simulink model "PlantaV4_2"  (R2021a)
settings: Solver=VariableStepAuto  StartTime=0.0  StopTime=60  MaxStep=1e-2  RelTol=1e-3
values from neighbouring files (symbols this model uses):
  alfahmax = ((2*ahmax)/(rhd))    (= 2)    [valoresPlanta_29_9_24.m]    (also in valoresPlanta_V3.m; valoresPlanta_v4.m)
  alfatmax = atmax/rtd    (= 1.6)    [valoresPlanta_29_9_24.m]    (also in valoresPlanta_V3.m; valoresPlanta_v4.m)
  atmax = 0.8    [valoresPlanta_29_9_24.m]    (also in valoresPlanta_V3.m; valoresPlanta_v4.m)
  ax_max = 0.8    [valoresPlanta_29_9_24.m]    (also in valoresPlanta_v4.m)
  ay_max = 0.75    [valoresPlanta_29_9_24.m]    (also in valoresPlanta_v4.m)
  bh_eq = bhm*ih^2+bhd    (= 8720)    [Valores.m]    (also in Valores_1.m; valoresPlanta.m; valoresPlanta_29_9_24.m; valoresPlanta_V3.m)
  bhb = 1e8    (= 100000000)    [Valores.m]    (also in Valores_1.m; valoresPlanta.m; valoresPlanta_29_9_24.m; valoresPlanta_V3.m)
  bhEb = 2.2e9    (= 2200000000)    [Valores.m]    (also in Valores_1.m; valoresPlanta.m; valoresPlanta_29_9_24.m; valoresPlanta_V3.m)
  bt = 90.0    (= 90)    [Valores.m]    (also in Valores_1.m; valoresPlanta.m; valoresPlanta_29_9_24.m; valoresPlanta_V3.m)
  bt_eq = btd+(btm*(it^2))    (= 5401.8)    [valoresPlanta.m]    (also in valoresPlanta_29_9_24.m; valoresPlanta_V3.m; valoresPlanta_v4.m)
  btw = 3.0e3    (= 3000)    [Valores.m]    (also in Valores_1.m; valoresPlanta.m; valoresPlanta_29_9_24.m; valoresPlanta_V3.m)
  bwu = 150    [Valores.m]    (also in Valores_1.m; valoresPlanta.m; valoresPlanta_29_9_24.m; valoresPlanta_V3.m)
  g = 9.80665    [Valores.m]    (also in Valores_1.m; valoresPlanta.m; valoresPlanta_29_9_24.m; valoresPlanta_V3.m)
  hMax = 10    [Valores_1.m]    (also in valoresPlanta.m; valoresPlanta_V3.m; valoresPlanta_v4.m)
  ih = 22    [Valores.m]    (also in Valores_1.m; valoresPlanta.m; valoresPlanta_29_9_24.m; valoresPlanta_V3.m)
  it = 30    [Valores.m]    (also in Valores_1.m; valoresPlanta.m; valoresPlanta_29_9_24.m; valoresPlanta_V3.m)
  Jh_eq = Jhm_hb*ih^2+Jhd_hEb    (= 18320)    [Valores.m]    (also in Valores_1.m; valoresPlanta.m; valoresPlanta_29_9_24.m; valoresPlanta_V3.m)
  Jt_eq = Jtd+(Jtm_tb*(it^2))    (= 7500)    [valoresPlanta.m]    (also in valoresPlanta_29_9_24.m; valoresPlanta_V3.m; valoresPlanta_v4.m)
  KDh = Jeq2 * w_posh^3    (= -12245.4404091)    [Valores.m]    (also in Valores_1.m = Jeq2 * w_posh; valoresPlanta.m = Jeq2 * w_posh; valoresPlanta_29_9_24.m = Jh_eq * n * w_posh; valoresPlanta_V3.m = Jeq2 * w_posh)
  KDt = Meq2 * w_post^3    (= -4728.86946035)    [Valores.m]    (also in Valores_1.m = Meq2 * w_post; valoresPlanta.m = Meq2 * w_post; valoresPlanta_29_9_24.m = 10127; valoresPlanta_V3.m = Meq2 * w_post)
  KIh = Jeq2 * w_posh^2    (= 2572.66592082)    [Valores.m]    (also in Valores_1.m = Jeq2 * w_posh^3; valoresPlanta.m = Jeq2 * w_posh^3; valoresPlanta_29_9_24.m = Jh_eq * w_posh^3; valoresPlanta_V3.m = Jeq2 * w_posh^3)
  KIt = Meq2 * w_post^2    (= 1307.690244)    [Valores.m]    (also in Valores_1.m = Meq2 * w_post^3; valoresPlanta.m = Meq2 * w_post^3; valoresPlanta_29_9_24.m = 6809.6; valoresPlanta_V3.m = Meq2 * w_post^3)
  KPh = Jeq2 * w_posh    (= -540.495867769)    [Valores.m]    (also in Valores_1.m = Jeq2 * w_posh^2; valoresPlanta.m = Jeq2 * w_posh^2; valoresPlanta_29_9_24.m = Jh_eq * n * w_posh^2; valoresPlanta_V3.m = Jeq2 * w_posh^2)
  KPt = Meq2 * w_post    (= -361.62)    [Valores.m]    (also in Valores_1.m = Meq2 * w_post^2; valoresPlanta.m = Meq2 * w_post^2; valoresPlanta_29_9_24.m = 14123; valoresPlanta_V3.m = Meq2 * w_post^2)
  Ktw = 4.8e5    (= 480000)    [Valores.m]    (also in Valores_1.m; valoresPlanta.m; valoresPlanta_29_9_24.m; valoresPlanta_V3.m)
  kwu = 2.36e8    (= 236000000)    [Valores.m]    (also in Valores_1.m; valoresPlanta.m; valoresPlanta_29_9_24.m; valoresPlanta_V3.m)
  Mc_max = 5e4    (= 50000)    [Valores.m]    (also in Valores_1.m; valoresPlanta.m; valoresPlanta_29_9_24.m; valoresPlanta_V3.m)
  Mc_min = 2e3    (= 2000)    [Valores.m]    (also in Valores_1.m; valoresPlanta.m; valoresPlanta_29_9_24.m; valoresPlanta_V3.m)
  Meq = Mt+(it^2*Jtm_tb+Jtd)/rtd^2    (= 60000)    [Valores.m]    (also in Valores_1.m; valoresPlanta_29_9_24.m; valoresPlanta_v4.m)
  Ms = 1.5e4    (= 15000)    [Valores.m]    (also in Valores_1.m; valoresPlanta.m; valoresPlanta_29_9_24.m; valoresPlanta_V3.m)
  Mt = 30000    [Valores.m]    (also in Valores_1.m; valoresPlanta.m; valoresPlanta_29_9_24.m; valoresPlanta_V3.m)
  pos = [p0; p1; p2; p3; p4; p5]    [calcularTrayectoria2_prueba.m]    (also in perfilObsaculos.m = puntosTrayectoria(4, 1.5, 20, [-20,0], estado_cont, hy_cont,; puntosTrayectoria.m; valoresPlanta_29_9_24.m = calcularTrayectoria2_prueba(vx_max, vhmax, ax_max, Hc, hx_co; valoresPlanta_v4.m = puntosTrayectoria(4, 1.5, 20, [-20,0], estado_cont, hy_cont,)
  rhd = 0.75    [Valores.m]    (also in Valores_1.m; valoresPlanta.m; valoresPlanta_29_9_24.m; valoresPlanta_V3.m)
  rtd = 0.5    [Valores.m]    (also in Valores_1.m; valoresPlanta.m; valoresPlanta_29_9_24.m; valoresPlanta_V3.m)
  tau_hm = 1e-3    (= 0.001)    [valoresPlanta.m]    (also in valoresPlanta_29_9_24.m; valoresPlanta_V3.m; valoresPlanta_v4.m)
  tau_tm = 1e-3    (= 0.001)    [Valores.m]    (also in Valores_1.m; valoresPlanta.m; valoresPlanta_29_9_24.m; valoresPlanta_V3.m)
  Thb_Max = 5e4    (= 50000)    [Valores.m]    (also in Valores_1.m; valoresPlanta.m; valoresPlanta_29_9_24.m; valoresPlanta_V3.m)
  ThEb_Max = 1.1e6    (= 1100000)    [Valores.m]    (also in Valores_1.m; valoresPlanta.m; valoresPlanta_29_9_24.m; valoresPlanta_V3.m)
  Thm_Max = 2e4    (= 20000)    [Valores.m]    (also in Valores_1.m; valoresPlanta.m; valoresPlanta_29_9_24.m; valoresPlanta_V3.m)
  Ttb_Max = 5e3    (= 5000)    [Valores.m]    (also in Valores_1.m; valoresPlanta.m; valoresPlanta_29_9_24.m; valoresPlanta_V3.m)
  Ttm_Max = 3e3    (= 3000)    [Valores.m]    (also in Valores_1.m; valoresPlanta.m; valoresPlanta_29_9_24.m = 4000; valoresPlanta_V3.m)
  v_x_max = 4    [Valores_1.m]    (also in valoresPlanta.m; valoresPlanta_V3.m = 0.4; valoresPlanta_v4.m)
  Yt0 = 45    [Valores.m]    (also in Valores_1.m; valoresPlanta.m; valoresPlanta_29_9_24.m; valoresPlanta_V3.m)
undefined symbols (not defined in the file or in its folder): sigbuilder_block
libraries: simulink_extras x1
settings Model: Creator=Matias  LastModifiedBy=agustin

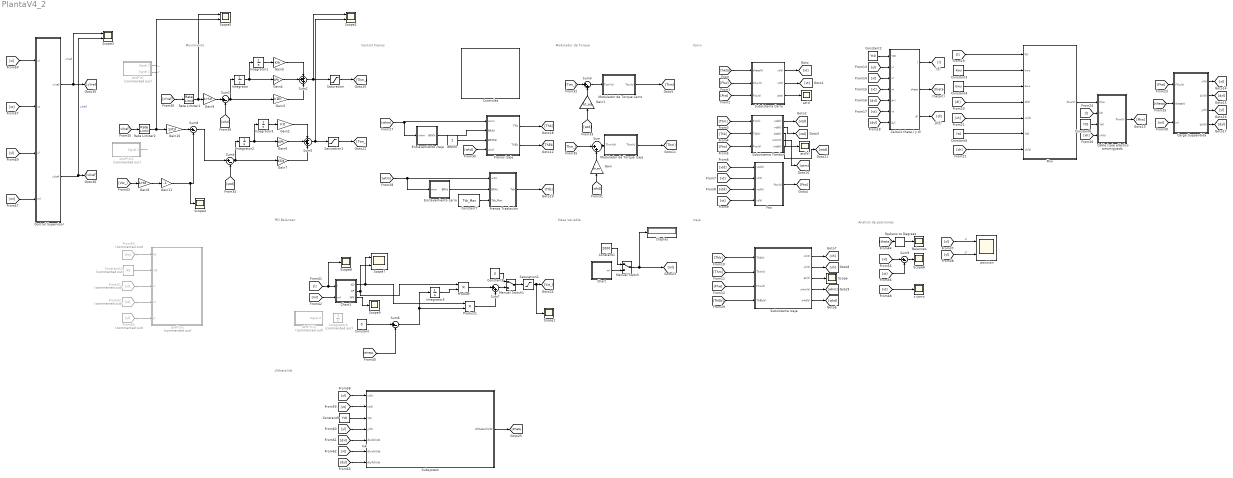
== system PlantaV4_2 ==
  note: d(theta)/dt
  note: Analisis de posiciones
  note: PID Balanceo
  note: Masa Variable
  note: Control Frenos
  note: Izaje
  note: Modulador de Torque
  note: Carro
  note: Movimiento
  In4 : Inport
  BRKhE : Constant
  Balanceo : Scope
  Cable izaje elástico amortiguado : Subsystem
  Calculo theta,l y dl : Subsystem
  Carga Suspendida : Subsystem
  Chart : Stateflow chart  TreatAsAtomicUnit=on
  Chart1 : Stateflow chart  TreatAsAtomicUnit=on
  Constant : Constant  Value=0
  Constant1 : Constant  Value=2000
  Constant12 : Constant  Commented=on  Value=45
  Constant{2,5..6,9} (4 alike) : Constant  Value=Yt0
  Constant3 : Constant  Value=kwu
  Constant4 : Constant  Value=bwu
  Constant7 : Constant  Value=Ttb_Max
  Constant8 : Constant  Value=0
  Control Supervisor : Subsystem
  Controles : Subsystem
  Display : Display
  Enclavamiento carro : Stateflow chart  TreatAsAtomicUnit=on
  Enclavamiento izaje : Stateflow chart  TreatAsAtomicUnit=on
  Fhw : Subsystem
  "Frenos Izaje " : Stateflow chart  TreatAsAtomicUnit=on
  Frenos Traslación : Stateflow chart  TreatAsAtomicUnit=on
  From51 : From  Commented=on  GotoTag=xl
  From52 : From  Commented=on  GotoTag=xt
  From53 : From  Commented=on  GotoTag=hc
  From54 : From  Commented=on  GotoTag=yl
  Ftw : Subsystem
  Gain : Gain  Gain=bh_eq
  Gain1 : Gain  Gain=bt_eq
  Gain10 : Gain  Gain=1/rtd
  Gain11 : Gain  Gain=.1
  Gain2 : Gain  Gain=KIt
  Gain3 : Gain  Gain=KDh
  Gain4 : Gain  Gain=KPh
  Gain5 : Gain  Gain=KIh
  Gain6 : Gain  Gain=KPt
  Gain7 : Gain  Gain=KDt
  Gain8 : Gain  Gain=1/rtd
  Gain9 : Gain  Gain=2/rhd
  Integrator{,1..3,5} (5 alike) : Integrator
  Integrator4 : Integrator  Commented=on
  Manual Switch : ManualSwitch
  Manual Switch1 : ManualSwitch
  Modulador de Torque Carro : Subsystem
  Modulador de Torque Izaje : Subsystem
  Product : Product
  Product1 : Product
  Radians to Degrees : simulink_extras/Transformations/Radians to Degrees
  Rate Limiter1 : RateLimiter  RisingSlewLimit=ay_max  FallingSlewLimit=-ay_max  SampleTimeMode=inherited
  Rate Limiter2 : RateLimiter  RisingSlewLimit=ax_max  FallingSlewLimit=-ax_max  SampleTimeMode=inherited
  Saturation : Saturate  UpperLimit=Thm_Max  LowerLimit=-Thm_Max
  Saturation1 : Saturate  UpperLimit=Ttm_Max  LowerLimit=-Ttm_Max
  Saturation2 : Saturate  UpperLimit=4  LowerLimit=-4
  Scope{,1,4,6,8..9} (6 alike) : Scope
  Scope{2..3,5,7} (4 alike) : Scope  NumInputPorts=2
  Subsistema Carro : Subsystem
  Subsistema Izaje : Subsystem
  Subsistema Tambor : Subsystem
  Subsystem : Subsystem
  Sum : Sum  Inputs=|++
  Sum{1,4,6,8..9} (5 alike) : Sum  Inputs=|+-
  Sum2 : Sum  Inputs=+++
  Sum3 : Sum  Inputs=|++
  Sum5 : Sum  Inputs=+++
  Sum7 : Sum  Inputs=|++
  at(t) : Scope
  atd(t) : Scope
  graficos : Stateflow chart  Commented=on  TreatAsAtomicUnit=on
  posicion : Scope  NumInputPorts=2
  whd*(t) : Subsystem  Tag=STV Subsys  Commented=on  LoadFcn=sigbuilder_block('load');  StartFcn=sigbuilder_block('start');  StopFcn=sigbuilder_block('stop');  ClipboardFcn=sigbuilder_block('clipboard');  mask(Sigbuilder block){tuvar=[0:10]}
      mask help: Simulink:masks:SigbuilderBlock_MD
      mask init:
      | if ~strcmp(get_param(bdroot(gcbh),'SimulationStatus'),'stopped') tuvar = sigbuilder_block('maskInit'); end
      settings: CopyFcn=sigbuilder_block('copy');  DeleteFcn=sigbuilder_block('delete');  ModelCloseFcn=sigbuilder_block('modelClose');  PreSaveFcn=sigbuilder_block('preSave');  PauseFcn=sigbuilder_block('pause');  ContinueFcn=sigbuilder_block('continue');  NameChangeFcn=sigbuilder_block('namechange');  OpenFcn=sigbuilder_block('open',[437.6 153 550.4 359.25 ]);  CloseFcn=sigbuilder_block('close');
      mask Display: plot(0, 0, 100, 100,[2, 2, 32, 32, 2], [68, 8, 8, 68, 68],[32, 2], [38, 38], [32, 19, 2],[53, 60, 44], [32, 17, 17, 2],[16, 16, 31, 31]);txt = getActiveGroup(gcbh);text(2, 100, txt,'verticalAlignment', 'top');
  whd*(t)1 : Subsystem  Tag=STV Subsys  Commented=on  LoadFcn=sigbuilder_block('load');  StartFcn=sigbuilder_block('start');  StopFcn=sigbuilder_block('stop');  ClipboardFcn=sigbuilder_block('clipboard');  mask(Sigbuilder block){tuvar=[0:10]}
      mask help: Simulink:masks:SigbuilderBlock_MD
      mask init:
      | if ~strcmp(get_param(bdroot(gcbh),'SimulationStatus'),'stopped') tuvar = sigbuilder_block('maskInit'); end
      settings: CopyFcn=sigbuilder_block('copy');  DeleteFcn=sigbuilder_block('delete');  ModelCloseFcn=sigbuilder_block('modelClose');  PreSaveFcn=sigbuilder_block('preSave');  PauseFcn=sigbuilder_block('pause');  ContinueFcn=sigbuilder_block('continue');  NameChangeFcn=sigbuilder_block('namechange');  OpenFcn=sigbuilder_block('open',[437.6 199.2 550.4 400 ]);  CloseFcn=sigbuilder_block('close');
      mask Display: plot(0, 0, 100, 100,[2, 2, 32, 32, 2], [68, 8, 8, 68, 68],[32, 2], [38, 38], [32, 19, 2],[53, 60, 44], [32, 17, 17, 2],[16, 16, 31, 31]);txt = getActiveGroup(gcbh);text(2, 100, txt,'verticalAlignment', 'top');
  whd*(t)2 : Subsystem  Tag=STV Subsys  Commented=on  LoadFcn=sigbuilder_block('load');  StartFcn=sigbuilder_block('start');  StopFcn=sigbuilder_block('stop');  ClipboardFcn=sigbuilder_block('clipboard');  mask(Sigbuilder block){tuvar=[0:10]}
      mask help: Simulink:masks:SigbuilderBlock_MD
      mask init:
      | if ~strcmp(get_param(bdroot(gcbh),'SimulationStatus'),'stopped') tuvar = sigbuilder_block('maskInit'); end
      settings: CopyFcn=sigbuilder_block('copy');  DeleteFcn=sigbuilder_block('delete');  ModelCloseFcn=sigbuilder_block('modelClose');  PreSaveFcn=sigbuilder_block('preSave');  PauseFcn=sigbuilder_block('pause');  ContinueFcn=sigbuilder_block('continue');  NameChangeFcn=sigbuilder_block('namechange');  OpenFcn=sigbuilder_block('open',[437.6 153 550.4 359.25 ]);  CloseFcn=sigbuilder_block('close');
      mask Display: plot(0, 0, 100, 100,[2, 2, 32, 32, 2], [68, 8, 8, 68, 68],[32, 2], [38, 38], [32, 19, 2],[53, 60, 44], [32, 17, 17, 2],[16, 16, 31, 31]);txt = getActiveGroup(gcbh);text(2, 100, txt,'verticalAlignment', 'top');
  x carro : Scope
  wires:
  Subsistema Tambor/1(xtd(t)) -> [xtd]
  Subsistema Tambor/2(vtd(t)) -> [vtd]
  Subsistema Carro/1(xt(t)) -> [xt]
  Subsistema Carro/2(vt(t)) -> [vt]
  Subsistema Carro/3(at(t)) -> at(t)/1
  Subsistema Tambor/3(atd(t)) -> atd(t)/1
  [Ttb] -> Subsistema Tambor/2(Ttb(t))
  [Ttm] -> Subsistema Tambor/1(Tm(t))
  [Ftw] -> Subsistema Carro/3(Ftw(t))
  [Fhw] -> Subsistema Carro/2(Fhw(t))
  [theta] -> Subsistema Carro/1(theta(t))
  [Ftw] -> Subsistema Tambor/3(Ftw(t))
  Ftw/1(Ftw(t)) -> [Ftw]
  [xtd] -> Ftw/1(xtd(t))
  [xt] -> Ftw/2(xt(t))
  [vtd] -> Ftw/3(vtd(t))
  [vt] -> Ftw/4(vt(t))
  Modulador de Torque Carro/1(Ttm(t)) -> [Ttm]
  [Thm] -> Subsistema Izaje/2(Thm(t))
  [Thb] -> Subsistema Izaje/1(Thb(t))
  [Fhw] -> Subsistema Izaje/3(Fhw(t))
  Subsistema Izaje/1(xh(t)) -> [xh]
  Subsistema Izaje/2(vh(t)) -> [vh]
  Subsistema Izaje/3(ah(t)) -> Scope/1
  Subsistema Izaje/4(whm(t)) -> [whm]
  Subsistema Tambor/4(wtm(t)) -> [wtm]
  Modulador de Torque Izaje/1(Thm(t)) -> [Thm]
  [dxl] -> Calculo theta,l y dl/5(dxl)
  Constant2/1 -> Calculo theta,l y dl/1(Yt0)
  [yl] -> Calculo theta,l y dl/2(yl)
  Calculo theta,l y dl/3(dl) -> [dl]
  Calculo theta,l y dl/1(l) -> [l]
  [dyl] -> Calculo theta,l y dl/7(dyl)
  [xl] -> Calculo theta,l y dl/3(xl)
  [vt] -> Calculo theta,l y dl/6(vt)
  [xt] -> Calculo theta,l y dl/4(xt)
  Calculo theta,l y dl/2(theta) -> [theta]
  [dl] -> Fhw/4(dl(t))
  [xh] -> Fhw/7(xh(t))
  Constant3/1 -> Fhw/2(kwu)
  [l] -> Fhw/1(l(t))
  Constant5/1 -> Fhw/6(Yt0)
  [vh] -> Fhw/5(vh(t))
  Constant4/1 -> Fhw/3(bwu)
  Fhw/1(Fhw(t)) -> Cable izaje elástico amortiguado/1(Fhw)
  [l] -> Cable izaje elástico amortiguado/2(l(t))
  Constant6/1 -> Cable izaje elástico amortiguado/3(Yt0)
  [xh] -> Cable izaje elástico amortiguado/4(xh(t))
  Cable izaje elástico amortiguado/1(Fhw(t)) -> [Fhw]
  [theta] -> Carga Suspendida/2(theta(t))
  [Fhw] -> Carga Suspendida/1(Fhw(t))
  Carga Suspendida/1(xl(t)) -> [xl]
  Carga Suspendida/4(dyl(t)) -> [dyl]
  Carga Suspendida/3(yl(t)) -> [yl]
  Carga Suspendida/2(dxl(t)) -> [dxl]
  [whm] -> "Frenos Izaje "/1(whm), Enclavamiento izaje/1(whm)
  [wtm] -> Enclavamiento carro/1(wtm), Frenos Traslación/1(wtm)
  Enclavamiento carro/1(BRKt) -> Frenos Traslación/2(BRKt)
  Enclavamiento izaje/1(BRKh) -> "Frenos Izaje "/2(BRKh)
  "Frenos Izaje "/2(ThEb) -> [ThEb]
  Constant7/1 -> Frenos Traslación/3(Ttb_Max)
  BRKhE/1 -> "Frenos Izaje "/3(BRKhE)
  "Frenos Izaje "/1(Thb) -> [Thb]
  Frenos Traslación/1(Ttb) -> [Ttb]
  Subsistema Izaje/5(whd(t)) -> [whd]
  [ThEb] -> Subsistema Izaje/4(ThEb(t))
  [whd] -> "Frenos Izaje "/4(whd)
  [Thm_] -> Sum/1
  Sum/1 -> Modulador de Torque Izaje/1(Thm*(t))
  [whd] -> Gain/1
  Gain/1 -> Sum/2
  Integrator1/1 -> Gain5/1
  Integrator/1 -> Integrator1/1, Gain4/1
  Sum1/1 -> Integrator/1, Gain3/1
  Gain4/1 -> Sum2/2
  Gain5/1 -> Sum2/1
  Gain3/1 -> Sum2/3
  Sum3/1 -> Modulador de Torque Carro/1(Ttm*(t))
  [Ttm_] -> Sum3/1
  Gain1/1 -> Sum3/2
  Subsistema Tambor/5(wtd(t)) -> [wtd]
  [wtd] -> Gain1/1
  Gain7/1 -> Sum5/3
  [wtd] -> Sum4/2
  Gain6/1 -> Sum5/2
  Gain2/1 -> Sum5/1
  Integrator2/1 -> Integrator3/1, Gain6/1
  Sum4/1 -> Gain7/1, Integrator2/1
  Integrator3/1 -> Gain2/1
  [xl] -> posicion/1  "xl"
  [yl] -> posicion/2  "yl"
  [whd] -> Sum1/2
  Manual Switch/1 -> Display/1, [ml]
  [ml] -> Carga Suspendida/3(ml)
  [l] -> Scope8/1, Chart1/1(l)
  [ml] -> Chart1/2(ml)
  Product/1 -> Sum7/1
  Product1/1 -> Sum7/2
  Sum6/1 -> Product1/2, Integrator5/1
  Chart1/1(KD) -> Scope7/1, Product1/1
  Chart1/2(KP) -> Product/1, Scope7/2
  Constant/1 -> Sum6/1
  Sum8/1 -> Sum4/1
  whd*(t)2/1(Signal 2) -> ?
  Sum7/1 -> Manual Switch1/2
  Chart/1(ml) -> Manual Switch/2
  Constant1/1 -> Manual Switch/1
  Constant8/1 -> Manual Switch1/1
  [yl] -> Control Supervisor/3(yl)
  Control Supervisor/2(vXref) -> Scope3/2, [vXref]  "vXref"
  Control Supervisor/1(vYref) -> Scope3/1, [vYref]  "vYref"
  [xl] -> Control Supervisor/1(xl)
  whd*(t)/2(Signal 1) -> ?
  whd*(t)/1(Signal 2) -> ?
  Gain9/1 -> Sum1/1
  Manual Switch1/1 -> Saturation2/1
  [ml] -> Control Supervisor/4(ml)
  Constant12/1 -> graficos/2(Yt0)
  From52/1 -> graficos/4(xt)
  From51/1 -> graficos/3(xl)
  From53/1 -> graficos/1(Hc)
  From54/1 -> graficos/5(yl)
  Sum2/1 -> Saturation/1, Scope2/1
  [xl] -> Sum9/1
  [xt] -> Sum9/2
  Sum9/1 -> Scope6/1
  [xt] -> x carro/1
  Radians to Degrees/1 -> Balanceo/1
  [theta] -> Radians to Degrees/1
  Chart1/3(WN) -> Scope9/1
  [dTheta] -> Sum6/2
  Integrator5/1 -> Product/2
  Gain8/1 -> Gain11/1
  Gain11/1 -> Sum8/2, Scope4/1
  [Vxt_] -> Gain8/1
  Sum5/1 -> Saturation1/1, Scope2/2
  Gain10/1 -> Sum8/1
  [xt] -> Control Supervisor/2(xt)
  [vYref] -> Rate Limiter1/1
  [vXref] -> Rate Limiter2/1
  [dyl] -> Subsystem/7(d(yl(t))/dt)
  [vt] -> Subsystem/6(d(xt(t))/dt)
  [dxl] -> Subsystem/5(d(xl(t))/dt)
  [yl] -> Subsystem/4(yl(t))
  [xt] -> Subsystem/2(xt(t))
  [xl] -> Subsystem/1(xl(t))
  Constant9/1 -> Subsystem/3(Yto)
  Subsystem/1(d(theta(t))/dt) -> [dTheta]
  Rate Limiter2/1 -> Gain10/1, Scope5/2
  Rate Limiter1/1 -> Scope5/1, Gain9/1
  Saturation2/1 -> Scope1/1, [Vxt_]
  Saturation/1 -> [Thm_]
  Saturation1/1 -> [Ttm_]

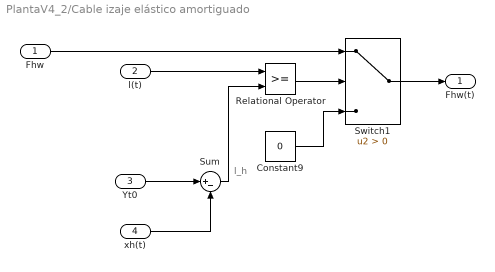
== system PlantaV4_2/Cable izaje elástico amortiguado ==
  note: l_h
  Fhw : Inport
  l(t) : Inport  Port=2
  Yt0 : Inport  Port=3
  xh(t) : Inport  Port=4
  Constant9 : Constant  Value=0
  Relational Operator : RelationalOperator  OutDataTypeStr=boolean  RndMeth=Simplest
  Sum : Sum  Inputs=|+-
  Switch1 : Switch  Criteria=u2 > Threshold
  Fhw(t) : Outport
  wires:
  l(t)/1 -> Relational Operator/1
  Sum/1 -> Relational Operator/2
  Fhw/1 -> Switch1/1
  Yt0/1 -> Sum/1
  Constant9/1 -> Switch1/3
  Relational Operator/1 -> Switch1/2
  xh(t)/1 -> Sum/2
  Switch1/1 -> Fhw(t)/1

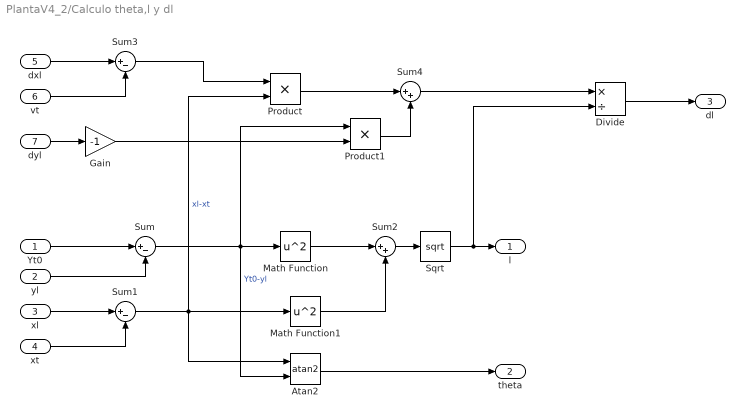
== system PlantaV4_2/Calculo theta,l y dl ==
  Yt0 : Inport
  yl : Inport  Port=2
  xl : Inport  Port=3
  xt : Inport  Port=4
  dxl : Inport  Port=5
  vt : Inport  Port=6
  dyl : Inport  Port=7
  Atan2 : Trigonometry  Operator=atan2
  Divide : Product  Inputs=*/
  Gain : Gain  Gain=-1
  Math Function : Math  Operator=square  SaturateOnIntegerOverflow=on
  Math Function1 : Math  Operator=square  SaturateOnIntegerOverflow=on
  Product : Product
  Product1 : Product
  Sqrt : Sqrt  SaturateOnIntegerOverflow=on
  Sum : Sum  Inputs=|+-
  Sum1 : Sum  Inputs=|+-
  Sum2 : Sum  Inputs=|++
  Sum3 : Sum  Inputs=|+-
  Sum4 : Sum  Inputs=|++
  l : Outport
  theta : Outport  Port=2
  dl : Outport  Port=3
  wires:
  Yt0/1 -> Sum/1
  yl/1 -> Sum/2
  xl/1 -> Sum1/1
  xt/1 -> Sum1/2
  Atan2/1 -> theta/1
  Sum1/1 -> Product/2, Math Function1/1, Atan2/1  "xl-xt"
  Sum/1 -> Product1/1, Atan2/2, Math Function/1  "Yt0-yl"
  Math Function/1 -> Sum2/1
  Math Function1/1 -> Sum2/2
  Sum2/1 -> Sqrt/1
  Sqrt/1 -> Divide/2, l/1
  dxl/1 -> Sum3/1
  vt/1 -> Sum3/2
  Sum3/1 -> Product/1
  dyl/1 -> Gain/1
  Gain/1 -> Product1/2
  Product/1 -> Sum4/1
  Product1/1 -> Sum4/2
  Sum4/1 -> Divide/1
  Divide/1 -> dl/1

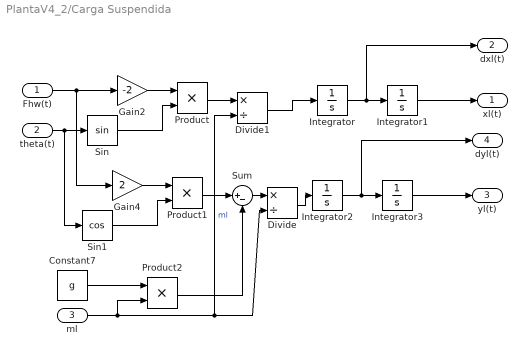
== system PlantaV4_2/Carga Suspendida ==
  Fhw(t) : Inport
  theta(t) : Inport  Port=2
  ml : Inport  Port=3
  Constant7 : Constant  Value=g
  Divide : Product  Inputs=*/
  Divide1 : Product  Inputs=*/
  Gain2 : Gain  Gain=-2
  Gain4 : Gain  Gain=2
  Integrator{,1..3} (4 alike) : Integrator
  Product : Product
  Product1 : Product
  Product2 : Product
  Sin : Trigonometry
  Sin1 : Trigonometry  Operator=cos
  Sum : Sum  Inputs=|+-
  xl(t) : Outport
  dxl(t) : Outport  Port=2
  yl(t) : Outport  Port=3
  dyl(t) : Outport  Port=4
  wires:
  Divide1/1 -> Integrator/1
  theta(t)/1 -> Sin1/1, Sin/1
  Constant7/1 -> Product2/1
  Product2/1 -> Sum/2
  Product/1 -> Divide1/1
  Fhw(t)/1 -> Gain4/1, Gain2/1
  Sum/1 -> Divide/1
  Integrator/1 -> dxl(t)/1, Integrator1/1
  Sin1/1 -> Product1/2
  Gain2/1 -> Product/1
  Product1/1 -> Sum/1
  Sin/1 -> Product/2
  Integrator1/1 -> xl(t)/1
  Integrator2/1 -> dyl(t)/1, Integrator3/1
  Divide/1 -> Integrator2/1
  Gain4/1 -> Product1/1
  Integrator3/1 -> yl(t)/1
  ml/1 -> Divide1/2, Divide/2, Product2/2  "ml"

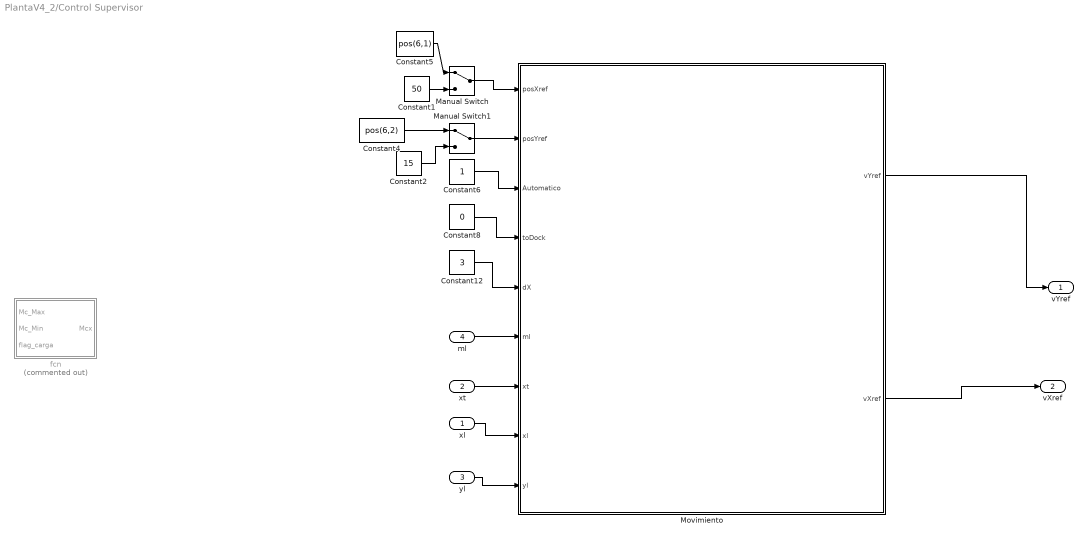
== system PlantaV4_2/Control Supervisor ==
  xl : Inport
  xt : Inport  Port=2
  yl : Inport  Port=3
  ml : Inport  Port=4
  Constant1 : Constant  Value=50
  Constant12 : Constant  Value=3
  Constant2 : Constant  Value=15
  Constant4 : Constant  Value=pos(6,2)
  Constant5 : Constant  Value=pos(6,1)
  Constant6 : Constant
  Constant8 : Constant  Value=0
  Manual Switch : ManualSwitch
  Manual Switch1 : ManualSwitch
  Movimiento : Stateflow chart  TreatAsAtomicUnit=on
      settings: PortSchema="{\"entries\":[{\"content\":{\"sides\":[{\"content\":{\"connectorIds\":[\"In1\",\"In2\",\"In3\",\"In4\",\"In7\",\"In8\",\"In9\",\"In5\",\"In6\"]},\"type\":\"ConnectorPlacement.EquallySpacedRectSide\",\"uuid\":\"7754e6e1-1487-4c5e-b93c-5b95548dc503\"},{\"content\":{\"connectorIds\":[\"Out1\",\"Out2\"],\"side\":\"RIGHT\"},\"type\":\"ConnectorPlacement.EquallySpacedRectSide\",\"uuid\":\"e49bdf6e-b30d-4ce2-b56a-406d79434d70\"},{\"content\":{\"connectorIds\":[],\"side\":\"TOP\"},\"type\":\"ConnectorPlacement.EquallySpacedRectSide\",\"uuid\":\"816dde99-88b4-4e51-8e7c-8334ef27840c\"}]},\"type\":\"ConnectorPlacement.EquallySpacedConnector\",\"uuid\":\"e43ca6b0-ace3-4be2-8389-da1b8832a6a4\"}],\"packageUris\":[\"http://schema.mathworks.com/mf0/Connector/R2020b\"],\"version\":\"1.0\"}"
  fcn : MATLAB Function  Commented=on  TreatAsAtomicUnit=on
  vYref : Outport
  vXref : Outport  Port=2
  wires:
  Manual Switch/1 -> Movimiento/1(posXref)
  Manual Switch1/1 -> Movimiento/2(posYref)
  Constant6/1 -> Movimiento/3(Automatico)
  Constant8/1 -> Movimiento/4(toDock)
  Constant12/1 -> Movimiento/7(dX)
  xl/1 -> Movimiento/5(xl)
  yl/1 -> Movimiento/6(yl)
  ml/1 -> Movimiento/8(ml)
  Movimiento/2(vXref) -> vXref/1
  Movimiento/1(vYref) -> vYref/1
  xt/1 -> Movimiento/9(xt)
  Constant5/1 -> Manual Switch/1
  Constant4/1 -> Manual Switch1/1
  Constant1/1 -> Manual Switch/2
  Constant2/1 -> Manual Switch1/2

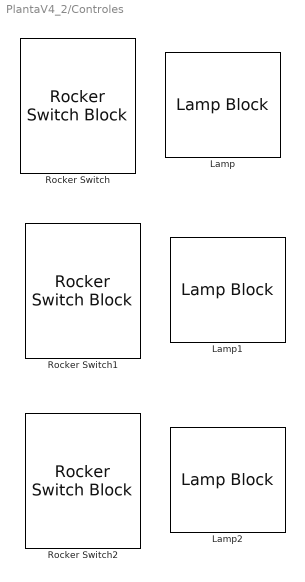
== system PlantaV4_2/Controles ==
  Lamp : LampBlock
  Lamp1 : LampBlock
  Lamp2 : LampBlock
  Rocker Switch : RockerSwitchBlock
      settings: Values={{'Off', 'On'}, [0 1]}
  Rocker Switch1 : RockerSwitchBlock
      settings: Values={{'Off', 'On'}, [0 1]}
  Rocker Switch2 : RockerSwitchBlock
      settings: Values={{'Off', 'On'}, [0 1]}

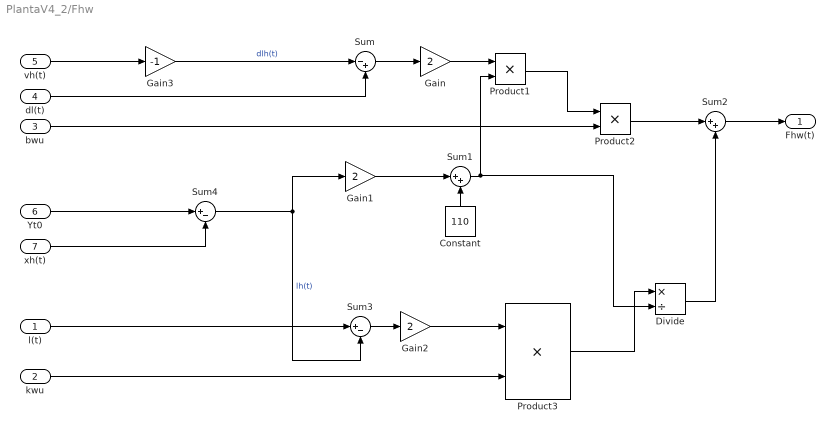
== system PlantaV4_2/Fhw ==
  l(t) : Inport
  kwu : Inport  Port=2
  bwu : Inport  Port=3
  dl(t) : Inport  Port=4
  vh(t) : Inport  Port=5
  Yt0 : Inport  Port=6
  xh(t) : Inport  Port=7
  Constant : Constant  Value=110
  Divide : Product  Inputs=*/
  Gain : Gain  Gain=2
  Gain1 : Gain  Gain=2
  Gain2 : Gain  Gain=2
  Gain3 : Gain  Gain=-1
  Product1 : Product
  Product2 : Product
  Product3 : Product
  Sum : Sum  Inputs=|-+
  Sum1 : Sum  Inputs=|++
  Sum2 : Sum  Inputs=|++
  Sum3 : Sum  Inputs=|+-
  Sum4 : Sum  Inputs=|+-
  Fhw(t) : Outport
  wires:
  dl(t)/1 -> Sum/2
  Sum/1 -> Gain/1
  Gain1/1 -> Sum1/1
  Sum4/1 -> Sum3/2, Gain1/1  "lh(t)"
  l(t)/1 -> Sum3/1
  Constant/1 -> Sum1/2
  Gain/1 -> Product1/1
  Sum1/1 -> Product1/2, Divide/2
  Product1/1 -> Product2/1
  bwu/1 -> Product2/2
  Product2/1 -> Sum2/1
  Sum3/1 -> Gain2/1
  Gain2/1 -> Product3/1
  kwu/1 -> Product3/2
  Product3/1 -> Divide/1
  Divide/1 -> Sum2/2
  Sum2/1 -> Fhw(t)/1
  vh(t)/1 -> Gain3/1
  Gain3/1 -> Sum/1  "dlh(t)"
  Yt0/1 -> Sum4/1
  xh(t)/1 -> Sum4/2

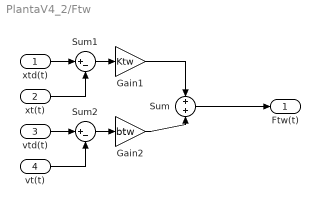
== system PlantaV4_2/Ftw ==
  xtd(t) : Inport
  xt(t) : Inport  Port=2
  vtd(t) : Inport  Port=3
  vt(t) : Inport  Port=4
  Gain1 : Gain  Gain=Ktw
  Gain2 : Gain  Gain=btw
  Sum : Sum
  Sum1 : Sum  Inputs=|+-
  Sum2 : Sum  Inputs=|+-
  Ftw(t) : Outport
  wires:
  Sum2/1 -> Gain2/1
  xtd(t)/1 -> Sum1/1
  vt(t)/1 -> Sum2/2
  xt(t)/1 -> Sum1/2
  Sum/1 -> Ftw(t)/1
  vtd(t)/1 -> Sum2/1
  Gain2/1 -> Sum/2
  Gain1/1 -> Sum/1
  Sum1/1 -> Gain1/1

== system PlantaV4_2/Modulador de Torque Carro ==
  Ttm*(t) : Inport
  Gain1 : Gain  Gain=1/tau_tm
  Integrator : Integrator
  Sum : Sum  Inputs=|+-
  Ttm(t) : Outport
  wires:
  Gain1/1 -> Integrator/1
  Integrator/1 -> Ttm(t)/1, Sum/2
  Ttm*(t)/1 -> Sum/1
  Sum/1 -> Gain1/1

== system PlantaV4_2/Modulador de Torque Izaje ==
  Thm*(t) : Inport
  Gain1 : Gain  Gain=1/tau_hm
  Integrator : Integrator
  Sum : Sum  Inputs=|+-
  Thm(t) : Outport
  wires:
  Gain1/1 -> Integrator/1
  Integrator/1 -> Thm(t)/1, Sum/2
  Thm*(t)/1 -> Sum/1
  Sum/1 -> Gain1/1

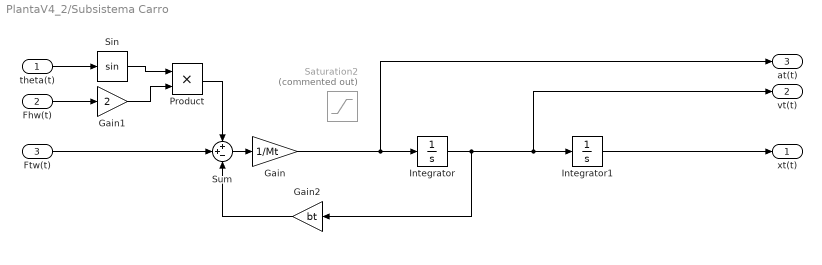
== system PlantaV4_2/Subsistema Carro ==
  theta(t) : Inport
  Fhw(t) : Inport  Port=2
  Ftw(t) : Inport  Port=3
  Gain : Gain  Gain=1/Mt
  Gain1 : Gain  Gain=2
  Gain2 : Gain  Gain=bt
  Integrator : Integrator
  Integrator1 : Integrator
  Product : Product
  Saturation2 : Saturate  Commented=on  UpperLimit=atmax  LowerLimit=-atmax
  Sin : Trigonometry
  Sum : Sum  Inputs=++-
  xt(t) : Outport
  vt(t) : Outport  Port=2
  at(t) : Outport  Port=3
  wires:
  Integrator/1 -> vt(t)/1, Integrator1/1, Gain2/1
  Gain1/1 -> Product/2
  theta(t)/1 -> Sin/1
  Sum/1 -> Gain/1
  Product/1 -> Sum/1
  Integrator1/1 -> xt(t)/1
  Ftw(t)/1 -> Sum/2
  Gain2/1 -> Sum/3
  Fhw(t)/1 -> Gain1/1
  Sin/1 -> Product/1
  Gain/1 -> at(t)/1, Integrator/1

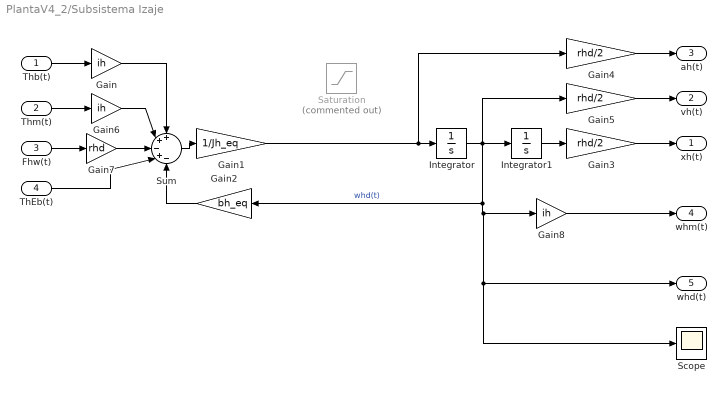
== system PlantaV4_2/Subsistema Izaje ==
  Thb(t) : Inport
  Thm(t) : Inport  Port=2
  Fhw(t) : Inport  Port=3
  ThEb(t) : Inport  Port=4
  Gain : Gain  Gain=ih
  Gain1 : Gain  Gain=1/Jh_eq
  Gain2 : Gain  Gain=bh_eq
  Gain3 : Gain  Gain=rhd/2
  Gain4 : Gain  Gain=rhd/2
  Gain5 : Gain  Gain=rhd/2
  Gain6 : Gain  Gain=ih
  Gain7 : Gain  Gain=rhd
  Gain8 : Gain  Gain=ih
  Integrator : Integrator
  Integrator1 : Integrator
  Saturation : Saturate  Commented=on  UpperLimit=alfahmax  LowerLimit=-alfahmax
  Scope : Scope
  Sum : Sum  Inputs=++-+-
  xh(t) : Outport
  vh(t) : Outport  Port=2
  ah(t) : Outport  Port=3
  whm(t) : Outport  Port=4
  whd(t) : Outport  Port=5
  wires:
  Integrator/1 -> Gain5/1, Integrator1/1, Scope/1, whd(t)/1, Gain8/1, Gain2/1  "whd(t)"
  Gain2/1 -> Sum/5
  Gain4/1 -> ah(t)/1
  Gain3/1 -> xh(t)/1
  Gain5/1 -> vh(t)/1
  Fhw(t)/1 -> Gain7/1
  Integrator1/1 -> Gain3/1
  Thb(t)/1 -> Gain/1
  Gain1/1 -> Gain4/1, Integrator/1
  Sum/1 -> Gain1/1
  Thm(t)/1 -> Gain6/1
  Gain/1 -> Sum/1
  Gain6/1 -> Sum/2
  Gain7/1 -> Sum/3
  ThEb(t)/1 -> Sum/4
  Gain8/1 -> whm(t)/1

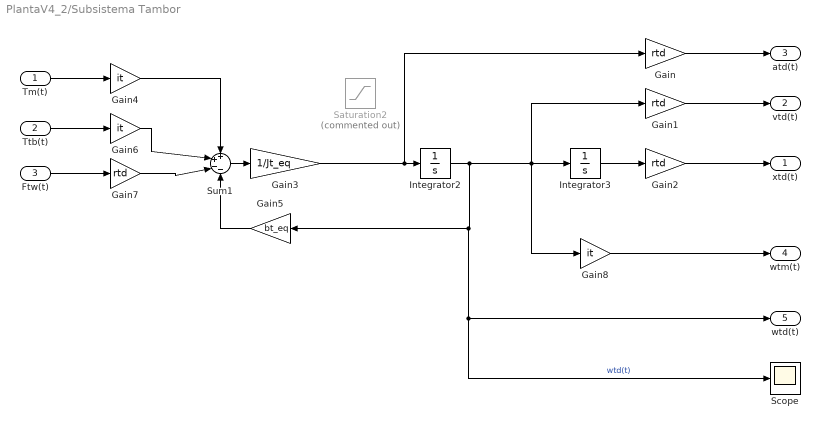
== system PlantaV4_2/Subsistema Tambor ==
  Tm(t) : Inport
  Ttb(t) : Inport  Port=2
  Ftw(t) : Inport  Port=3
  Gain{,1..2,7} (4 alike) : Gain  Gain=rtd
  Gain3 : Gain  Gain=1/Jt_eq
  Gain4 : Gain  Gain=it
  Gain5 : Gain  Gain=bt_eq
  Gain6 : Gain  Gain=it
  Gain8 : Gain  Gain=it
  Integrator2 : Integrator
  Integrator3 : Integrator
  Saturation2 : Saturate  Commented=on  UpperLimit=alfatmax  LowerLimit=-alfatmax
  Scope : Scope
  Sum1 : Sum  Inputs=++--
  xtd(t) : Outport
  vtd(t) : Outport  Port=2
  atd(t) : Outport  Port=3
  wtm(t) : Outport  Port=4
  wtd(t) : Outport  Port=5
  wires:
  Integrator3/1 -> Gain2/1
  Ftw(t)/1 -> Gain7/1
  Gain2/1 -> xtd(t)/1
  Integrator2/1 -> Gain8/1, Gain1/1, Integrator3/1, Scope/1, wtd(t)/1, Gain5/1  "wtd(t)"
  Tm(t)/1 -> Gain4/1
  Ttb(t)/1 -> Gain6/1
  Sum1/1 -> Gain3/1
  Gain5/1 -> Sum1/4
  Gain1/1 -> vtd(t)/1
  Gain/1 -> atd(t)/1
  Gain4/1 -> Sum1/1
  Gain6/1 -> Sum1/2
  Gain7/1 -> Sum1/3
  Gain8/1 -> wtm(t)/1
  Gain3/1 -> Gain/1, Integrator2/1

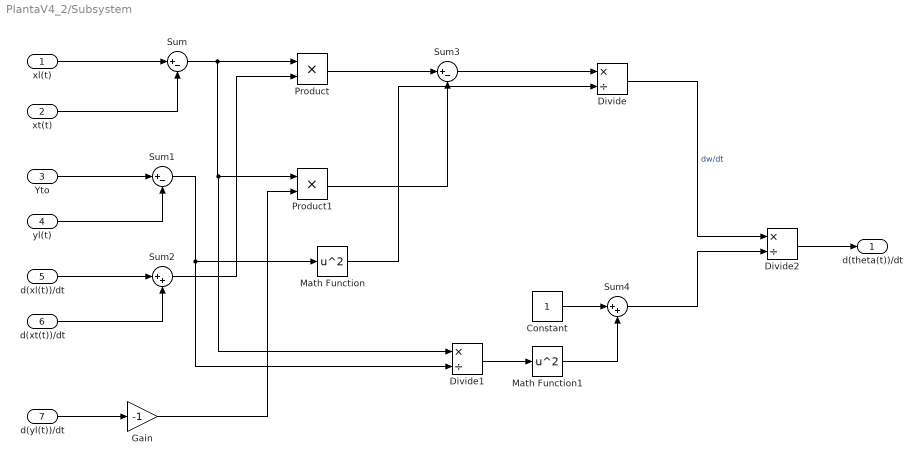
== system PlantaV4_2/Subsystem ==
  xl(t) : Inport
  xt(t) : Inport  Port=2
  Yto : Inport  Port=3
  yl(t) : Inport  Port=4
  d(xl(t))/dt : Inport  Port=5
  d(xt(t))/dt : Inport  Port=6
  d(yl(t))/dt : Inport  Port=7
  Constant : Constant
  Divide : Product  Inputs=*/
  Divide1 : Product  Inputs=*/
  Divide2 : Product  Inputs=*/
  Gain : Gain  Gain=-1
  Math Function : Math  Operator=square  SaturateOnIntegerOverflow=on
  Math Function1 : Math  Operator=square  SaturateOnIntegerOverflow=on
  Product : Product
  Product1 : Product
  Sum : Sum  Inputs=|+-
  Sum1 : Sum  Inputs=|+-
  Sum2 : Sum  Inputs=|++
  Sum3 : Sum  Inputs=|+-
  Sum4 : Sum  Inputs=|++
  d(theta(t))/dt : Outport
  wires:
  xl(t)/1 -> Sum/1
  xt(t)/1 -> Sum/2
  Yto/1 -> Sum1/1
  yl(t)/1 -> Sum1/2
  Sum/1 -> Divide1/1, Product1/1, Product/1
  d(xl(t))/dt/1 -> Sum2/1
  d(xt(t))/dt/1 -> Sum2/2
  Sum2/1 -> Product/2
  Product/1 -> Sum3/1
  Product1/1 -> Sum3/2
  d(yl(t))/dt/1 -> Gain/1
  Gain/1 -> Product1/2
  Sum3/1 -> Divide/1
  Sum1/1 -> Math Function/1, Divide1/2
  Math Function/1 -> Divide/2
  Divide/1 -> Divide2/1  "dw/dt"
  Divide1/1 -> Math Function1/1
  Math Function1/1 -> Sum4/2
  Constant/1 -> Sum4/1
  Divide2/1 -> d(theta(t))/dt/1
  Sum4/1 -> Divide2/2

== system PlantaV4_2/whd*(t) ==
  Demux : Demux  Tag=STV Demux  Outputs=2
      settings: DisplayOption=none
  FromWs : FromWorkspace  Tag=STV FromWs  VariableName=tuvar
      SigBuilderData=|
      | common.afterFinalStr = 'Extrapolate'
      | common.sampleTime = 0
      | dataSet.timeRange = [0 100]
      | dataSet.name = 'Group 1'
      | sbobj.Groups.Name = 'Group 1'
      | sbobj.Groups.Signals(1).Name = 'Signal 2'
      | sbobj.Groups.Signals(1).XData = [0 10 20 25 60 100]
      | sbobj.Groups.Signals(1).YData = [0 1 0.65 0.29 0 0]
      | sbobj.Groups.Signals(2).Name = 'Signal 1'
      | sbobj.Groups.Signals(2).XData = [0 40 40 60 60 100]
      | sbobj.Groups.Signals(2).YData = [0 0 1 1 0 0]
      | sbobj.Groups.TimeRange = [0 100]
  Signal 2 : Outport  Tag=STV Outport
  Signal 1 : Outport  Tag=STV Outport  Port=2
  wires:
  FromWs/1 -> Demux/1
  Demux/1 -> Signal 2/1
  Demux/2 -> Signal 1/1

== system PlantaV4_2/whd*(t)1 ==
  Demux : Demux  Tag=STV Demux  Outputs=1
      settings: DisplayOption=none
  FromWs : FromWorkspace  Tag=STV FromWs  VariableName=tuvar
      SigBuilderData=|
      | common.afterFinalStr = 'Extrapolate'
      | common.sampleTime = 0
      | dataSet.timeRange = [0 100]
      | dataSet.name = 'Group 1'
      | sbobj.Groups.Name = 'Group 1'
      | sbobj.Groups.Signals.Name = 'Signal 2'
      | sbobj.Groups.Signals.XData = [0 10 20 25 60 100]
      | sbobj.Groups.Signals.YData = [0 1 1 0 0 0]
      | sbobj.Groups.TimeRange = [0 100]
  Signal 2 : Outport  Tag=STV Outport
  wires:
  FromWs/1 -> Demux/1
  Demux/1 -> Signal 2/1

== system PlantaV4_2/whd*(t)2 ==
  Demux : Demux  Tag=STV Demux  Outputs=1
      settings: DisplayOption=none
  FromWs : FromWorkspace  Tag=STV FromWs  VariableName=tuvar
      SigBuilderData=|
      | common.afterFinalStr = 'Extrapolate'
      | common.sampleTime = 0
      | dataSet.timeRange = [0 100]
      | dataSet.name = 'Group 1'
      | sbobj.Groups.Name = 'Group 1'
      | sbobj.Groups.Signals.Name = 'Signal 2'
      | sbobj.Groups.Signals.XData = [0 10 20 25 60 100]
      | sbobj.Groups.Signals.YData = [0 0.1 0.1 0 0 0]
      | sbobj.Groups.TimeRange = [0 100]
  Signal 2 : Outport  Tag=STV Outport
  wires:
  FromWs/1 -> Demux/1
  Demux/1 -> Signal 2/1

== stateflow chart PlantaV4_2/Frenos Traslación ==
  state FrenosOperacion
    state BRKt_off
      during:
      Ttb=-btb*wtm;
      Ttb=min(Ttb_Max,max(-Ttb_Max, Ttb));
    state BRKt_on
      during:
      Ttb=0;
    (default) -> BRKt_off
    BRKt_off -> BRKt_on : [BRKt==1 ]
    BRKt_on -> BRKt_off : [BRKt==0]
  data: Ttb output; wtm input; btb parameter; BRKt input; Ttb_Max input

== stateflow chart PlantaV4_2/Chart ==
  state Masa
    entry:
    ml = fcn(Mc_max, Mc_min);
  data: Mc_MAX function_input; Mc_MIN function_input; ML function_output; Mc_max parameter; ml output; Mc_min parameter; flag_carga local
  function ML = fcn(Mc_MAX, Mc_MIN):
    | function ML = fcn(Mc_MAX, Mc_MIN)
    | %Agregar: sobrecarga
    | %if (flag_carga == 1)
    |     ML = Mc_MIN + (Mc_MAX - Mc_MIN)*rand(1);
    |     %ml = Mc_Max + 0.01 * randi([1,15],1) * Mc_Max;
    | %else
    |  %   ML = 0;
    | %end
    | end

== stateflow chart PlantaV4_2/Frenos Izaje  ==
  state FrenosOperacion
    state BRKh_off
      during:
      Thb=-bhb*whm;
      Thb=min(Thb_Max,max(-Thb_Max,Thb ));
    state BRKh_on
      during:
      Thb=0;
    (default) -> BRKh_off
    BRKh_off -> BRKh_on [order 1] : [BRKh==1 && BRKhE==1]
    BRKh_on -> BRKh_off [order 1] : [BRKh==0 && BRKhE==1]
  state FrenosEmergencia
    state BRKhE_off
      during:
      ThEb=-bhEb*whd;
      ThEb=min(ThEb_Max,max(-ThEb_Max, ThEb));
    state BRKhE_on
      during:
      ThEb=0;
    (default) -> BRKhE_off
    BRKhE_off -> BRKhE_on : [BRKhE==1]
    BRKhE_on -> BRKhE_off [order 1] : [BRKhE==0]
  BRKh_on -> FrenosEmergencia [order 2] : [BRKhE==0]
  BRKh_off -> FrenosEmergencia [order 2] : [BRKhE==0]
  BRKhE_on -> FrenosOperacion [order 2] : [BRKhE==1]
  (default) -> FrenosEmergencia
  data: whm input; bhb parameter; BRKh input; bhEb parameter; BRKhE input; Thb output; ThEb output; Thb_Max parameter; ThEb_Max parameter; whd input

== stateflow chart PlantaV4_2/Chart1 ==
  state Balanceo
    during:
    [KP,KD, WN]=balanceo(Meq, Mt,ml,l,g)
  (default) -> Balanceo
  data: MEQ function_input; mt function_input; Ml function_input; Kd function_output; Kp function_output; L function_input; G function_input; wn function_output; l input; ml input; KD output; KP output; g parameter; Meq parameter; WN output; Mt parameter
  function [Kd,Kp, wn]=balanceo(MEQ, mt,Ml,L,G):
    | function [Kd,Kp, wn]=balanceo(MEQ, mt,Ml,L,G)
    |     
    | %     Kd=(1+(L*(mt+Ml)))/(mt+Ml);
    | %     Kp=(2*0.7*wn)/(mt+Ml);
    | %     w=((mt*G/((mt+Ml)*L))^0.5);
    | %     Kd=(mt*G/w^2 + (mt+Ml)*L)/(Ml+mt);
    | %     Kp=2*0.7*(-(mt+Ml)*L/(Ml+mt)+Kd);
    |     
    |     %correccion agustin
    |     %wn=((mt*G)/(L*(mt+Ml)))^(0.5);
    |     %Kd = L - (mt*G)/((mt+Ml)*wn^2);
    |     %Kp = (2*z*wn)/(L-Kd);
    |     %correcion matias
    |     z = 0.9;
    |     wn=((MEQ*G)/(L*(MEQ+Ml)))^(0.5);
    |     wn = 2 * wn; %el mejor: 2
    |     Kd = ((-MEQ*G)/(wn^2) +(MEQ+Ml)*L)* 1/(mt+Ml);
    |     Kp = ((2*z*wn)*((MEQ+Ml)* L - Kd*(mt+Ml)))/(mt+Ml);
    | end

== stateflow chart PlantaV4_2/Enclavamiento carro ==
  (default) -> (junction 9) : % activacion de frenos
  (junction 9) -> (junction 4) [order 1] : [abs(wtm)<wtmMax]
  (junction 9) -> (junction 10) [order 2] : {BRKt=0;}
  (junction 4) -> (junction 2) : {BRKt=1;}
  (junction 2) -> (junction 10)
  (junction 10) -> (junction 11)
  data: wtmMax parameter; wtm input; BRKt output

== stateflow chart PlantaV4_2/Enclavamiento izaje ==
  (default) -> (junction 9) : % activacion de frenos
  (junction 9) -> (junction 4) [order 1] : [abs(whm)<whmMax]
  (junction 9) -> (junction 10) [order 2] : {BRKh=0;}
  (junction 4) -> (junction 2) : {BRKh=1;}
  (junction 2) -> (junction 10)
  (junction 10) -> (junction 11)
  data: whm input; BRKh output; whmMax parameter

== stateflow chart PlantaV4_2/graficos ==
  state Graficar
    entry:
    cont = 0;
    %contenedor = rectangle('Position',[xl-2.25, yl, 4.5, 2.5 ],'FaceColor','g');
    %carro = rectangle('Position',[xt-2, Yt0, 4.5, 2 ],'FaceColor','r');
    during:
    dock_shore_graph(xt, xl, yl, Yt0,Hc,cont);
    cont = cont+1;
  (default) -> Graficar
  data: Xt function_input; Xl function_input; Yl function_input; YT0 function_input; HC function_input; Con function_input; Hc input; Yt0 input; xl input; xt input; yl input; cont local
  function dock_shore_graph(Xt, Xl, Yl, YT0, HC,Con):
    | function dock_shore_graph(Xt, Xl, Yl, YT0, HC,Con)
    | %viga voladiza
    | plot([-30 50],[45 45 ],'Color','k')
    | hold on
    | %cable
    | cable = plot([xt xl],[45 yl+Hc],'Color','k');
    | %carro (modificar luego)
    | carro = rectangle('Position',[xt-2, Yt0, 4.5, 2 ],'FaceColor','r');
    | %Conenedor
    | contenedor = rectangle('Position',[xl-2.25, yl, 4.5, 2.5 ],'FaceColor','g');
    | %barco
    | rectangle('Position',[2, -20.5, 0.5, 25.5 ],'FaceColor','b');
    | rectangle('Position',[50, -20.5, 0.5, 25.5 ],'FaceColor','b');
    | rectangle('Position',[2, -20.5, 48, 0.5 ],'FaceColor','b');
    | %muelle
    | rectangle('Position',[-30, -0.5, 30, 0.5 ],'FaceColor','k');
    | rectangle('Position',[0, -20, 0.5, 20 ],'FaceColor','k');
    | 
    | title("Operacion de carga y descarga");
    | xlabel("Distancia (mts)");
    | ylabel("Altura (mts)");
    | hold on
    | if (cont>0)
    |     set(carro, 'Position', [xt-2, Yt0, 4.5, 2 ]);
    |     set(contenedor, 'Position', [xl-2.25, yl, 4.5, 2.5 ]);
    |     set(cable,'XData', [xt xl], 'YData', [45 yl]);
    |     %cable = plot([xt xl],[45 yl],'Color','k');
    | end
    | % %perfil de contenedores VARIABLE
    | % x = 6.5:5:46.5;
    | % y = [15 20 32 16 35 11 32 22 10];
    | % b = bar(x,y); %,'histc'
    | % b(1).BaseValue = -20;
    | % b(1).BaseLine.LineWidth = 0.01;
    | % b(1).ShowBaseLine=0;
    | % b(1).BarWidth=0.9;
    | % b(1).FaceColor = [0.8500 0.3250 0.0980];
    | % % Actualizar los datos del gráfico de barras
    | % set(b, 'YData', datos);
    | %---------------------------------------------------
    | % Perfil de contenedores
    | puntos_iniciales = [5 -20; 10 -20; 15 -20; 20 -20; 25 -20; 30 -20; 35 -20; 40 -20; 45 -20];
    | % Definir las dimensiones de los rectángulos
    | dimensiones = [15; 12; 20; 18; 14; 16; 13; 10; 8];
    | 
    | % Bucle para crear los rectángulos
    | for i = 1:size(puntos_iniciales, 1)
    |     % Obtener las coordenadas del punto inicial
    |     x = puntos_iniciales(i, 1);
    |     y = puntos_iniciales(i, 2);
    |     altura = dimensiones(i);
    |     % Crear el rectángulo utilizando el comando 'rectangle'
    |     rectangle('Position', [x, y, 5, altura], 'FaceColor', 'red');
    |     
    | %     hold on; % Para mantener los rectángulos en el gráfico
    | end
    | 
    | % Refrescar el gráfico
    | drawnow;
    | 
    | % Pausa para observar el cambio en el gráfico
    | pause(0.5);
    | set(carro, 'visible', 'off');
    | set(contenedor, 'visible', 'off');
    | set(cable, 'visible', 'off');
    | % if (mod(cont,7)==0)
    | %     set(carro, 'visible', 'off');
    | %     set(contenedor, 'visible', 'off');
    | %     %carro (modificar luego)
    | % carro = rectangle('Position',[xt-2, Yt0, 4.5, 2 ],'FaceColor','r');
    | % %Conenedor
    | % contenedor = rectangle('Position',[xl-2.25, yl, 4.5, 2.5 ],'FaceColor','g');
    | % end
    | end

== stateflow chart PlantaV4_2/Control Supervisor/Movimiento ==
  state estado_inicial [commented out]
    entry:
    vYref = 0;
    vXref = 0;
    flag_carga = 1;
  state Movimiento [commented out]
    entry:
    h_i = 0;
    h_seg = 0;
    %[h_i, h_seg] = calculaH1(v_x_max, dX, hMax, v_y_max,dh);
    %v_x_max = 4;
    during:
    v_y_max = calcVel(ml, g);
    %v_y_max = 2;
    h_i = 5;
    h_seg = 15;
    %[h_i, h_seg] = calculaH1(v_x_max, dX, hMax, v_y_max,dh);
    state Estado4 [commented out]
      entry:
      E = 4; %estado 4
      during:
      if (toDock==1)
      vYref = v_y_max; %suma
      vXref = v_x_max;  %cte desaceleracion hasta 0 (suma)
      else
      vYref = v_y_max; %suma
      vXref = 0.1;  %cte desaceleracion hasta 0
      end
    state Estado3 [commented out]
      entry:
      E = 3; %estado 3
      during:
      vYref = 0;
      if (toDock==1)
      vXref = -v_x_max;
      else
      vXref = v_x_max;
      end
    state Estado2 [commented out]
      entry:
      E = 2; %estado 2
      during:
      if (toDock==1)
      vYref = -v_y_max;
      vXref = -v_x_max;
      else
      vYref = v_y_max;
      vXref = v_x_max;
      end
    note: %ver de comparar con posicion objetivo
        | definir hmax (2 contenedores)
    state DescargaConteiner [commented out]
      entry:
      ml = Ms;
    state Estado5 [commented out]
      entry:
      E = 5; %estado 5
      during:
      if (toDock==1)
      vYref = vYref+0.5; %acelero
      vXref = 0;
      %ml = Ms;
      else
      vYref = vYref-0.5; %desacelero
      vXref = 0;
      end
    state Estado1 [commented out]
      entry:
      E = 1; %estado 1
      during:
      if (toDock==1)
      if (yl > 0)
      vYref = -v_y_max;
      end
      else
      vYref = v_y_max;
      if (yl < h_i)
      vYref = 0;
      end
      end
    state EstadoInicial [commented out]
      entry:
      entry:
      E = 0; %estado 0
      vYref = 0;
      vXref = 0;
      flag_carga = 0;
      ml = fcn(Mc_Max, Mc_Min);
    Estado3 -> Estado2 [commented out] : [xl<=dX && toDock==1 && yl >= h_seg]
    Estado3 -> Estado4 [commented out] : [xl>= posXref-7.5 && toDock==0]
    Estado2 -> Estado3 [commented out] : [xl>=dX && toDock==0 && yl >= h_seg]
    Estado4 -> Estado3 [commented out] : [xl<= posXref-7.5 && toDock==1]
    Estado4 -> Estado5 [commented out] : [yl==hMax && vXref<=0 && toDock==0]
    Estado5 -> Estado4 [commented out] : [yl==hMax && toDock==1]
    Estado2 -> Estado1 [commented out] : [yl<=h_i && toDock==1]
    Estado1 -> Estado2 [commented out] : [yl >= h_i && toDock==0]
    Estado5 -> DescargaConteiner [commented out] : [yl == posYref && toDock==0]
    DescargaConteiner -> EstadoInicial [commented out] : [Automatico == 1 && flag_carga == 1]
    (default) -> EstadoInicial [commented out]
    EstadoInicial -> Estado1 [commented out] : [Automatico == 1 && toDock==0]
    EstadoInicial -> Estado5 [commented out] : [Automatico == 1 && toDock==1]
    Estado1 -> EstadoInicial [commented out] : [Automatico == 1 && toDock==1]
  state estado_inicial1
    entry:
    vYref = 0;
    vXref = 0;
    flag_carga = 1;
  state Manual [commented out]
  state Movimiento1
    entry:
    h_i = 0;
    h_seg = 25;
    v_y_max = calcVel(ml, g); %que la v no se pase de vmaxima
    %v_y_max = 0.75; %solo de prueba: valores de aceleracion
    during:
    %v_y_max = 1;
    h_i = 0;
    %h_i = pos(1,1);
    %h_seg = pos(3,2);
    h_seg = 45;
    state e6
      entry:
      vXref = v_x_max;
      during:
      vYref = 0;
      if (xl>posXref*0.85)
      vXref = v_x_max*0.5;
      elseif (xl>posXref*0.8)
      vXref = v_x_max*0.6;
      elseif (xl>posXref*0.70)
      vXref = v_x_max*0.75;
      end
    state e4
      entry:
      vYref = v_y_max;
      during:
      % ------------------
      if (yl>h_seg*0.85)
      vYref = v_y_max*0.5;
      vXref = v_x_max*0.75;
      elseif (yl>h_seg*0.8)
      vYref = v_y_max*0.6;
      vXref = v_x_max*0.6;
      elseif (yl>h_seg*0.75)
      vYref = v_y_max*0.75;
      vXref = v_x_max*0.5;
      end
    state e2
      during:
      vXref = v_x_max;
      vYref = 0
    state e5
      entry:
      vXref = vXref;
      during:
      vXref = v_x_max*0.45;
      vYref = -v_y_max;
    state e1
      during:
      vXref = 0;
      vYref = v_y_max;
      if (yl<h_seg*0.15)
      vYref = v_y_max*0.25;
      elseif (yl<h_seg*0.30)
      vYref = v_y_max*0.5;
      elseif (yl<h_seg*0.45)
      vYref = v_y_max*0.75;
      else
      vYref = v_y_max;
      end
    state e3
      entry:
      vYref = -v_y_max;
      %vXref = v_x_max;
      during:
      vXref = vXref*0.5;
      vYref = -v_y_max
    state e01
      during:
      vXref = 0;
      vYref = 0;
    state e0
      during:
      vXref = 0;
      vYref = 0;
    e2 -> e6 : [(xl>posXref*0.75) && toDock==0]
    e4 -> e2 : [(yl>=h_seg) && toDock==0]
    e6 -> e5 : [(xl>posXref*0.9) && toDock==0]
    e1 -> e4 : [(yl>h_seg*0.75) && toDock==0]
    e5 -> e3 : [(xt>=posXref*0.98) && toDock==0]
    e3 -> e01 : [(yl<=posYref) && toDock==0]
    e0 -> e1 : [toDock==0 ]
    (default) -> e0
    (default) -> ? [commented out] : [(yl<posYref+0.2) && toDock==0]
  (default) -> estado_inicial [commented out]
  estado_inicial -> Manual [commented out] : [Automatico == 0]
  estado_inicial -> Movimiento [commented out] : [Automatico == 1]
  (default) -> estado_inicial1
  Movimiento -> Manual [commented out] : [Automatico == 0]
  Manual -> Movimiento [commented out] : [Automatico == 1]
  estado_inicial1 -> Movimiento1 : [Automatico == 1]
  data: VXmax function_input; DX function_input; HMax function_input; HIni function_output; HSeg function_output; VYmax function_input; Dh function_input; Ml function_input; vMaxY function_output; G function_input; ML function_output; Mc_MAX function_input; Mc_MIN function_input; VXmax function_input; DX function_input; HMax function_input; HIni function_output; HSeg function_output; VYmax function_input; Dh function_input; Ml function_input; vMaxY function_output; G function_input; posXref input; posYref input; Automatico input =1; v_y_max local; toDock input; xl input; yl input; v_x_max parameter; dX input =15; hMax parameter; h_i local; h_seg local; g parameter; Ms parameter; E local; vYref output; vXref output; flag_carga local; ml input; xt input; pos parameter
  function [HIni, HSeg] = calculaH1(VXmax, DX, HMax, VYmax,Dh):
    | function [HIni, HSeg] = calculaH1(VXmax, DX, HMax, VYmax,Dh)
    |     t = VXmax/DX;   %tiempo necesario para llegar del p inicial al barco
    |     hp = t * VYmax;  %altura de mayor pendiente posible
    |     HSeg = HMax + Dh;   %máxima altura de contenedores + altura operativa
    |     HIni = hSeg - hp;
    | end
  function vMaxY = calcVel(Ml, G):
    | function vMaxY = calcVel(Ml, G)
    |  vMaxY = 956.15e3/((Ml)*G);
    | end
  function ML = fcn(Mc_MAX, Mc_MIN):
    | function ML = fcn(Mc_MAX, Mc_MIN)
    | %Agregar: sobrecarga
    | if (flag_carga == 1)
    |     ML = Mc_MIN + (Mc_MAX - Mc_MIN)*rand(1);
    |     %ml = Mc_Max + 0.01 * randi([1,15],1) * Mc_Max;
    | else
    |     ML = 0;
    | end
    | end
  function [HIni, HSeg] = calculaH1(VXmax, DX, HMax, VYmax,Dh):
    | function [HIni, HSeg] = calculaH1(VXmax, DX, HMax, VYmax,Dh)
    |     t = VXmax/DX;   %tiempo necesario para llegar del p inicial al barco
    |     hp = t * VYmax;  %altura de mayor pendiente posible
    |     HSeg = HMax + Dh;   %máxima altura de contenedores + altura operativa
    |     HIni = hSeg - hp;
    | end
  function vMaxY = calcVel(Ml, G):
    | function vMaxY = calcVel(Ml, G)
    | %falta corregir para que no choque a una velocidad menor 
    | v = 956.15e3/((Ml)*G);
    |  if (v > 4)
    |      vMaxY = 4;
    |  else
    |      vMaxY = v;
    |  end
    | end

== matlab function PlantaV4_2/Control Supervisor/fcn ==
  data: Mc_Max input; Mcx output; Mc_Min input; flag_carga input
function Mcx = fcn(Mc_Max, Mc_Min, flag_carga)
%Agregar: sobrecarga
if (flag_carga == 1)
    Mcx = Mc_Min + (Mc_Max - Mc_Min)*rand(1);
    %ml = Mc_Max + 0.01 * randi([1,15],1) * Mc_Max;
else
    Mcx = 0;
end
end
